simulink model "Equiv_compact_therm_network_of_IGBT_modules_heat_sink_systm"  (R2015a)
settings: Solver=ode45  StartTime=0.0  StopTime=10.0  RelTol=1e-3
libraries: fl_lib x15
settings Model: Creator=Caner  LastModifiedBy=Caner

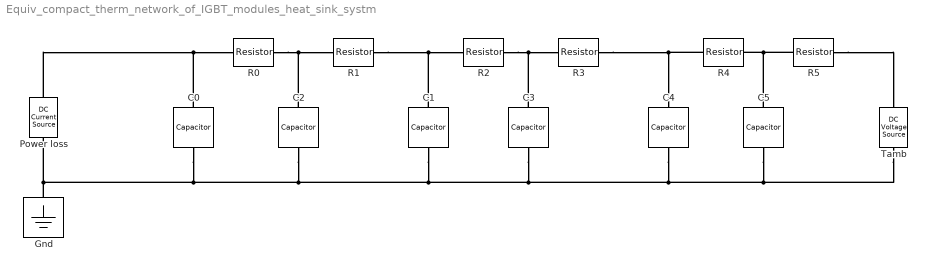
== system Equiv_compact_therm_network_of_IGBT_modules_heat_sink_systm ==
  C{0..2,4} (4 alike) : fl_lib/Electrical/Electrical Elements/Capacitor  c=1e-6 F  r=1e-6 Ohm  g=0 1/Ohm  i_specify=off  i_priority=High  i=0 A  v_specify=off  v_priority=High  v=0 V  vc_specify=off  vc_priority=High  vc=0 V
  "C3 " : fl_lib/Electrical/Electrical Elements/Capacitor  c=1e-6 F  r=1e-6 Ohm  g=0 1/Ohm  i_specify=off  i_priority=High  i=0 A  v_specify=off  v_priority=High  v=0 V  vc_specify=off  vc_priority=High  vc=0 V
  "C5 " : fl_lib/Electrical/Electrical Elements/Capacitor  c=1e-6 F  r=1e-6 Ohm  g=0 1/Ohm  i_specify=off  i_priority=High  i=0 A  v_specify=off  v_priority=High  v=0 V  vc_specify=off  vc_priority=High  vc=0 V
  Gnd : fl_lib/Electrical/Electrical Elements/Electrical Reference
  Power loss : fl_lib/Electrical/Electrical Sources/DC Current Source  i0=1 A
  R{0..5} (6 alike) : fl_lib/Electrical/Electrical Elements/Resistor  R=1 Ohm  i_specify=off  i_priority=High  i=0 A  v_specify=off  v_priority=High  v=0 V
  Tamb : fl_lib/Electrical/Electrical Sources/DC Voltage Source  v0=1 V
  connections:
  Power loss/LConn1 -- R0/LConn1 -- C0/LConn1
  R0/RConn1 -- R1/LConn1 -- C2/LConn1
  R1/RConn1 -- C1/LConn1 -- R2/LConn1
  R2/RConn1 -- "C3 "/LConn1 -- R3/LConn1
  R3/RConn1 -- R4/LConn1 -- C4/LConn1
  R5/LConn1 -- "C5 "/LConn1 -- R4/RConn1
  R5/RConn1 -- Tamb/LConn1
  Gnd/LConn1 -- Tamb/RConn1 -- "C5 "/RConn1 -- C4/RConn1 -- "C3 "/RConn1 -- C1/RConn1 -- C2/RConn1 -- C0/RConn1 -- Power loss/RConn1
